simulink model "esp32_receiver"  (R2025a)
settings: Solver=FixedStepDiscrete  StartTime=0.0  StopTime=5  FixedStep=1/fs  RelTol=1e-3
values from neighbouring files (symbols this model uses):
  fs = 8000    [init_receiver.m]    (also in tx_signal.m; tx_workspace.mat)
settings Model: Creator=Subham Sarkar  LastModifiedBy=Subham Sarkar

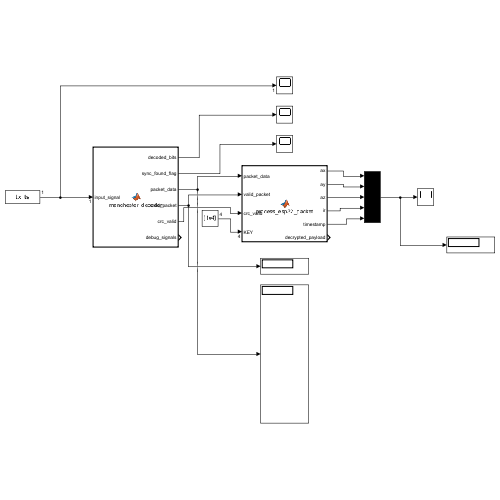
[thumbnail: Simulink's stored preview of the top-level diagram]
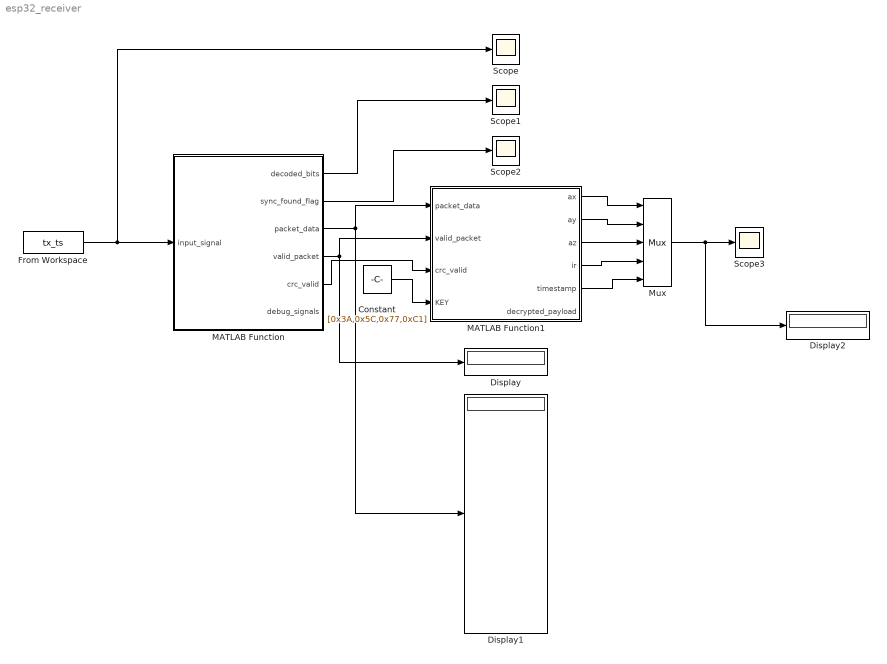
== system esp32_receiver ==
  Constant : Constant  Value=[0x3A,0x5C,0x77,0xC1]
  Display : Display
  Display1 : Display
  Display2 : Display
  From Workspace : FromWorkspace  VariableName=tx_ts  SampleTime=1/fs
  MATLAB Function : MATLAB Function  TreatAsAtomicUnit=on
  MATLAB Function1 : MATLAB Function  TreatAsAtomicUnit=on
  Mux : Mux  Inputs=5
  Scope{,1..3} (4 alike) : Scope
      Scope settings: ActiveDisplayYMinimum=-0.0865691131491112  ActiveDisplayYMaximum=1.1039070773270789
      Scope1 settings: ActiveDisplayYMinimum=-0.865153177289626  ActiveDisplayYMaximum=0.862522019773326
      Scope2 settings: ActiveDisplayYMinimum=-1  ActiveDisplayYMaximum=1  DataLoggingVariableName=ScopeData2
      Scope3 settings: ActiveDisplayYMinimum=-0.9094169112992323  ActiveDisplayYMaximum=0.853529022454586  DataLoggingVariableName=ScopeData3
  wires:
  From Workspace/1 -> Scope/1, MATLAB Function/1(input_signal)
  MATLAB Function/3(packet_data) -> Display1/1, MATLAB Function1/1(packet_data)
  MATLAB Function/4(valid_packet) -> Display/1, MATLAB Function1/2(valid_packet)
  MATLAB Function/1(decoded_bits) -> Scope1/1
  MATLAB Function/2(sync_found_flag) -> Scope2/1
  Constant/1 -> MATLAB Function1/4(KEY)
  MATLAB Function1/1(ax) -> Mux/1
  MATLAB Function1/2(ay) -> Mux/2
  MATLAB Function1/3(az) -> Mux/3
  MATLAB Function1/4(ir) -> Mux/4
  MATLAB Function1/5(timestamp) -> Mux/5
  Mux/1 -> Display2/1, Scope3/1
  MATLAB Function/5(crc_valid) -> MATLAB Function1/3(crc_valid)

== matlab function esp32_receiver/MATLAB Function1 ==
  data: packet_data input; ax output; valid_packet input; crc_valid input; KEY input; ay output; az output; ir output; timestamp output; decrypted_payload output
function [ax, ay, az, ir, timestamp, decrypted_payload] = process_esp32_packet(packet_data, valid_packet, crc_valid, KEY)
% Process ESP32 packet data and extract sensor values

% Initialize outputs with proper types
ax = double(0); 
ay = double(0); 
az = double(0); 
ir = double(0); 
timestamp = double(0);
decrypted_payload = zeros(1, 0, 'uint8');

if valid_packet && crc_valid && length(packet_data) >= 5
    len = double(packet_data(5));
    if length(packet_data) >= (5 + len + 1)
        payload_enc = packet_data(6:5+len);
        
        % Decrypt payload
        decrypted_payload = alu_decrypt_bytes(payload_enc, KEY);
        
        % Extract sensor data (big-endian)
        if length(decrypted_payload) >= 11
            % Calculate timestamp as uint32 first, then convert to double
            timestamp_uint32 = bitshift(uint32(decrypted_payload(1)), 24) + ...
                              bitshift(uint32(decrypted_payload(2)), 16) + ...
                              bitshift(uint32(decrypted_payload(3)), 8) + ...
                              uint32(decrypted_payload(4));
            timestamp = double(timestamp_uint32);
            
            % Extract accelerometer values
            ax_int16 = typecast(uint8([decrypted_payload(5), decrypted_payload(6)]), 'int16');
            ay_int16 = typecast(uint8([decrypted_payload(7), decrypted_payload(8)]), 'int16');
            az_int16 = typecast(uint8([decrypted_payload(9), decrypted_payload(10)]), 'int16');
            
            ax = double(ax_int16);
            ay = double(ay_int16);
            az = double(az_int16);
            ir = double(decrypted_payload(11));
        end
    end
end
end

== matlab function esp32_receiver/MATLAB Function ==
  data: input_signal input; decoded_bits output; sync_found_flag output; packet_data output; valid_packet output; crc_valid output; debug_signals output
function [decoded_bits, sync_found_flag, packet_data, valid_packet, crc_valid, debug_signals] = manchester_decoder(input_signal)
%#codegen

% Parameters
SYNC_WORD = uint32(hex2dec('AAAAAA2D'));
MAX_BITS = 1024;
persistent bitstream bit_count in_sync packet_buffer packet_index

if isempty(bitstream)
    bitstream = false(1, MAX_BITS);
    bit_count = uint32(0);
    in_sync = false;
    packet_buffer = false(1, MAX_BITS);
    packet_index = uint32(0);
end

decoded_bits = false(1, MAX_BITS);
sync_found_flag = false;
packet_data = zeros(1, 100, 'uint8');
valid_packet = false;
crc_valid = false;

% Step 1: Manchester pair decoding
persistent man_buf man_cnt debug_man_buf debug_bit_val debug_word_val debug_sync_match
if isempty(man_buf)
    man_buf = false(1,2);
    man_cnt = uint8(0);
    debug_man_buf = false(1,2);
    debug_bit_val = false;
    debug_word_val = uint32(0);
    debug_sync_match = false;
end

% Signal conditioning - simple filtering and thresholding
persistent filter_buf
if isempty(filter_buf)
    filter_buf = false(1, 3);
end

for k = 1:length(input_signal)
    % Signal conditioning
    filter_buf = [filter_buf(2:3), input_signal(k)];
    conditioned_signal = mean(double(filter_buf)) > 0.5;
    
    % Accumulate pairs
    man_cnt = man_cnt + 1;
    man_buf(man_cnt) = conditioned_signal;
    debug_man_buf = man_buf;

    if man_cnt == 2
        man_cnt = uint8(0);

        % Decode valid pairs - try both conventions
        if man_buf(1)==1 && man_buf(2)==0
            bit_val = true;      % Convention 1: 1->[1 0]
        elseif man_buf(1)==0 && man_buf(2)==1
            bit_val = false;     % Convention 1: 0->[0 1]
        else
            % Try opposite convention
            if man_buf(1)==0 && man_buf(2)==1
                bit_val = true;  % Convention 2: 0->1 means logic 1
            elseif man_buf(1)==1 && man_buf(2)==0
                bit_val = false; % Convention 2: 1->0 means logic 0
            else
                % invalid pair → skip
                continue;
            end
        end
        
        debug_bit_val = bit_val;

        % Shift register for sync detection
        bit_count = bit_count + 1;
        if bit_count > MAX_BITS
            bit_count = uint32(1);
        end
        bitstream(bit_count) = bit_val;

        % Convert last 32 bits into integer
        if bit_count >= 32
            word_val = uint32(0);
            for i = 0:31
                if bit_count > i
                    bit_val_temp = bitstream(bit_count - i);
                else
                    bit_val_temp = false;
                end
                word_val = bitor(word_val, bitshift(uint32(bit_val_temp), i));
            end
            debug_word_val = word_val;
            debug_sync_match = (word_val == SYNC_WORD);

            % Sync detection
            if ~in_sync && word_val == SYNC_WORD
                in_sync = true;
                sync_found_flag = true;
                packet_index = uint32(0);
                bit_count = uint32(0);
            end
        end

        % If in sync → store bits for packet processing
        if in_sync
            packet_index = packet_index + 1;
            if packet_index <= MAX_BITS
                packet_buffer(packet_index) = bit_val;
            end
            
            % Check if we have a complete packet (minimum 5 bytes: preamble+sync+len)
            if packet_index >= 40
                [packet_bytes, valid, crc_ok] = process_packet(packet_buffer(1:packet_index));
                if valid
                    packet_data(1:length(packet_bytes)) = packet_bytes;
                    valid_packet = true;
                    crc_valid = crc_ok;
                    in_sync = false;
                end
            end
        end
    end
end

% Output decoded bits for visualization
if packet_index > 0
    decoded_bits(1:min(MAX_BITS, packet_index)) = packet_buffer(1:min(MAX_BITS, packet_index));
end

% Debug signals output
debug_signals = struct(...
    'man_buf', debug_man_buf, ...
    'bit_val', debug_bit_val, ...
    'word_val', debug_word_val, ...
    'sync_match', debug_sync_match, ...
    'bit_count', double(bit_count), ...
    'packet_index', double(packet_index), ...
    'conditioned_signal', conditioned_signal ...
);

end

function [packet_bytes, valid, crc_ok] = process_packet(bits)
    % Convert bits to bytes
    num_bits = length(bits);
    num_bytes = floor(num_bits / 8);
    packet_bytes = zeros(1, num_bytes, 'uint8');
    valid = false;
    crc_ok = false;
    
    if num_bytes < 5  % Minimum: preamble(3) + sync(1) + len(1)
        return;
    end
    
    for i = 1:num_bytes
        byte_val = uint8(0);
        for j = 1:8
            bit_pos = (i-1)*8 + j;
            if bit_pos <= num_bits && bits(bit_pos)
                byte_val = bitor(byte_val, bitshift(1, 8-j));
            end
        end
        packet_bytes(i) = byte_val;
    end
    
    % Verify preamble and sync
    if packet_bytes(1) == 170 && packet_bytes(2) == 170 && packet_bytes(3) == 170 && packet_bytes(4) == 45
        valid = true;
        
        % Check CRC if we have enough bytes
        len = double(packet_bytes(5));
        if num_bytes >= (5 + len + 1)
            payload = packet_bytes(6:5+len);
            received_crc = packet_bytes(6+len);
            computed_crc = compute_crc8_mexstyle(payload);
            crc_ok = (received_crc == computed_crc);
        end
    end
end

function CRC = compute_crc8_mexstyle(data)
    % Simple CRC-8 (poly 0x07) — input: uint8 vector
    crc = uint8(0);
    for ii = 1:numel(data)
        crc = bitxor(crc, data(ii));
        for b=1:8
            if bitand(crc, 128)
                crc = bitxor( bitshift(crc,1,'uint8'), uint8(7) ); % poly 0x07
            else
                crc = bitshift(crc,1,'uint8');
            end
        end
    end
    CRC = crc;
end

function out = alu_decrypt_bytes(buf, KEY)
    % Decryption: reverse of encryption
    L = numel(buf);
    out = zeros(1,L,'uint8');
    for i=1:L
        k = KEY(mod(i-1,4)+1);
        b = buf(i);
        b1 = bitxor(b, uint8(i-1));
        b2 = uint8(mod(double(b1) - double(k) + 256, 256));
        b3 = bitxor(b2, k);
        out(i) = b3;
    end
end
